simulink model "sensors002"  (Simulink 8.3)
settings: Solver=ode45  StartTime=0.0  StopTime=10.0  RelTol=1e-3
settings Model: Creator=swami  LastModifiedBy=swami
settings DataIOCC: SignalLoggingSaveFormat=Dataset
settings DebuggingCC: UnderspecifiedInitializationDetection=Simplified  MergeDetectMultiDrivingBlocksExec=error  FrameProcessingCompatibilityMsg=error  StateNameClashWarn=none
settings GRTTargetCC: CombineOutputUpdateFcns=on  GRTInterface=off

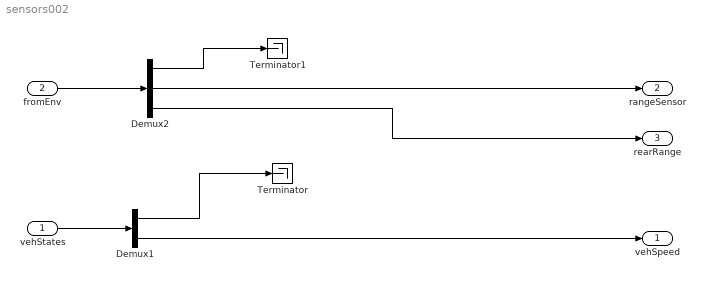
== system sensors002 ==
  vehStates : Inport
  fromEnv : Inport  Port=2
  Demux1 : Demux  Outputs=2
  Demux2 : Demux  Outputs=3
  Terminator : Terminator
  Terminator1 : Terminator
  vehSpeed : Outport
  rangeSensor : Outport  Port=2
  rearRange : Outport  Port=3
  wires:
  Demux1/1 -> Terminator/1
  Demux1/2 -> vehSpeed/1
  Demux2/1 -> Terminator1/1
  Demux2/2 -> rangeSensor/1
  Demux2/3 -> rearRange/1
  fromEnv/1 -> Demux2/1
  vehStates/1 -> Demux1/1
